simulink subsystem "rectified_dc"  (R2024a)
settings: Solver=VariableStepAuto  StartTime=0.0  StopTime=10.0  RelTol=1e-3
model mask{peak_voltage=100}
  mask prompts: peak_voltage "PeakVoltage"
libraries: spsDiodeLib x4, spsACVoltageSourceLib x1
settings Model: Creator=javeed  LastModifiedBy=javeed

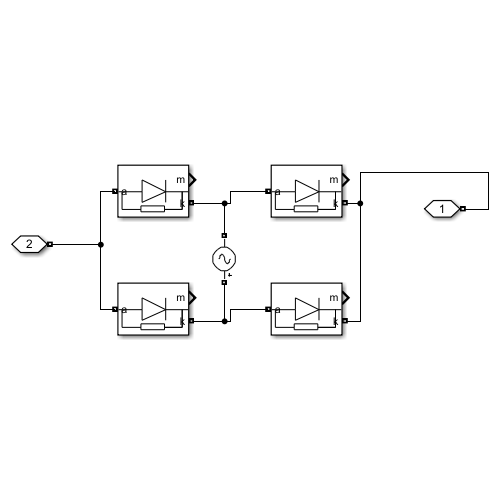
[thumbnail: Simulink's stored preview of the top-level diagram]
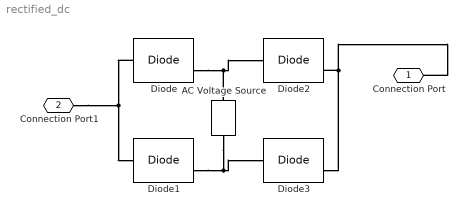
== system rectified_dc ==
  AC Voltage Source : spsACVoltageSourceLib/AC Voltage Source  Amplitude=peak_voltage  Phase=0  Frequency=50  SampleTime=0  Measurements=None  BusType=swing  Pref=10e3  Qref=0  Qmin=-inf  Qmax=+inf
  Diode{,1..3} (4 alike) : spsDiodeLib/Diode  Ron=0.001  Lon=0  Vf=0.8  IC=0  UseSnubber=0  Rs=500  Cs=250e-9  Measurements=on
  Connection Port : PMIOPort  Side=Right
  Connection Port1 : PMIOPort  Port=2  Side=Left
  connections:
  Diode/RConn1 -- Diode2/LConn1 -- AC Voltage Source/LConn1
  Diode/LConn1 -- Diode1/LConn1 -- Connection Port1/RConn1
  Diode1/RConn1 -- Diode3/LConn1 -- AC Voltage Source/RConn1
  Diode3/RConn1 -- Connection Port/RConn1 -- Diode2/RConn1
